simulink library "NNodeTether_cl"  (R2018b)
settings: Solver=VariableStepAuto  StartTime=0.0  StopTime=10.0  RelTol=1e-3
values from neighbouring files (symbols this model uses):
  numNodes = 2    [tether000Test_ts.m]    (also in tether000_init.m = evalin('base',get_param(gcb,'numNodes')))
libraries: nodeDragForce_ul x1, nodeNetBuoyForce_ul x1, nodeSpringDamperForce_ul x1
settings Model: Creator=mcobb  LastModifiedBy=M.Cobb

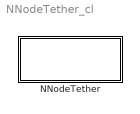
== system NNodeTether_cl ==
  NNodeTether : Subsystem

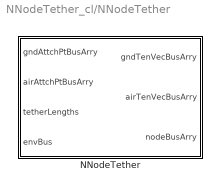
== system NNodeTether_cl/NNodeTether ==
  NNodeTether : Subsystem  mask{thr=0, flowDensity=10, gravity=0}
      mask prompts: thr "Tether Structure"; flowDensity "Fluid Density"; gravity "Gravitational Acceleration"

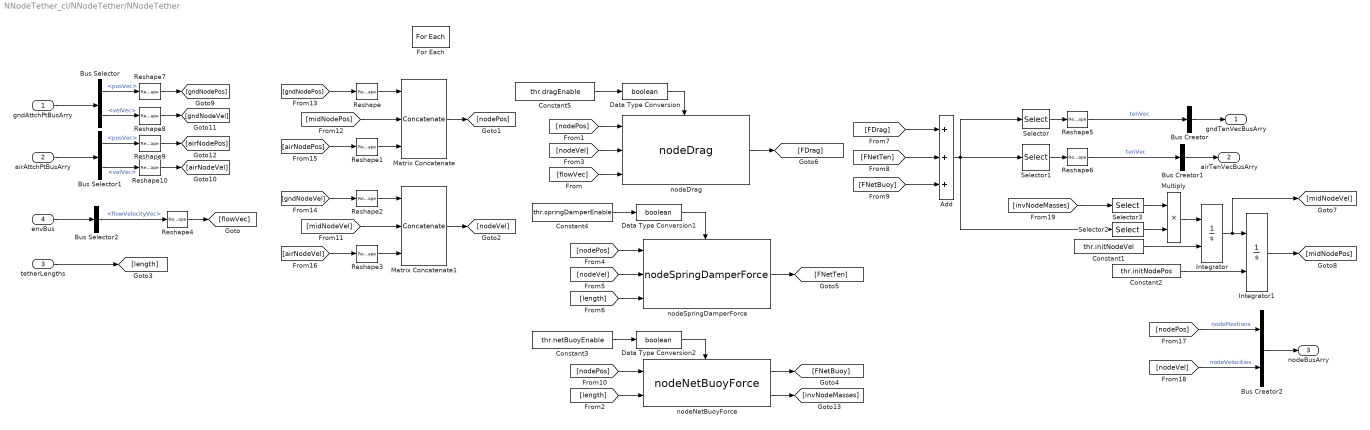
== system NNodeTether_cl/NNodeTether/NNodeTether ==
  gndAttchPtBusArry : Inport  OutDataTypeStr=Bus: thrAttachPtKinematicsBus  Partition=on  PartitionDimension=1  PartitionWidth=1  PartitionOffset=0
  airAttchPtBusArry : Inport  Port=2  OutDataTypeStr=Bus: thrAttachPtKinematicsBus  Partition=on  PartitionDimension=1  PartitionWidth=1  PartitionOffset=0
  tetherLengths : Inport  Port=3  Partition=on  PartitionDimension=1  PartitionWidth=1  PartitionOffset=0
  envBus : Inport  Port=4  OutDataTypeStr=Bus: envBus
  Add : Sum  Inputs=3
  Bus Creator : BusCreator  Inputs=1  OutDataTypeStr=Bus: thrTenVecBus  NonVirtualBus=on
  Bus Creator1 : BusCreator  Inputs=1  OutDataTypeStr=Bus: thrTenVecBus  NonVirtualBus=on
  Bus Creator2 : BusCreator  Inputs=2  OutDataTypeStr=Bus: thrNodeBus  NonVirtualBus=on
  Bus Selector : BusSelector  OutputSignals=posVec,velVec
  Bus Selector1 : BusSelector  OutputSignals=posVec,velVec
  Bus Selector2 : BusSelector  OutputSignals=flowVelocityVec
  Constant1 : Constant  Value=thr.initNodeVel
  Constant2 : Constant  Value=thr.initNodePos
  Constant3 : Constant  Value=thr.netBuoyEnable
  Constant4 : Constant  Value=thr.springDamperEnable
  Constant5 : Constant  Value=thr.dragEnable
  Data Type Conversion : DataTypeConversion  OutDataTypeStr=boolean
  Data Type Conversion1 : DataTypeConversion  OutDataTypeStr=boolean
  Data Type Conversion2 : DataTypeConversion  OutDataTypeStr=boolean
  For Each : ForEach  DisableCoverage=on  IterateSubsysMaskParameter=on,off,off  SubsysMaskParameterIterationDimension=2,1,1  IndexMode=One-based
  Integrator : Integrator  InitialConditionSource=external
  Integrator1 : Integrator  InitialConditionSource=external
  Matrix Concatenate : Concatenate  NumInputs=3  Mode=Multidimensional array  ConcatenateDimension=2
  Matrix Concatenate1 : Concatenate  NumInputs=3  Mode=Multidimensional array  ConcatenateDimension=2
  Multiply : Product
  Reshape{,1..10} (11 alike) : Reshape  OutputDimensionality=Column vector (2-D)
  Selector : Selector  NumberOfDimensions=2  InputPortWidth=3  IndexOptions=Select all,Index vector (dialog)  Indices=[1 3],1  OutputSizes=1,1
  Selector1 : Selector  NumberOfDimensions=2  InputPortWidth=3  IndexOptions=Select all,Starting index (dialog)  Indices=[1 3],numNodes  OutputSizes=1,1
  Selector2 : Selector  NumberOfDimensions=2  InputPortWidth=3  IndexOptions=Select all,Index vector (dialog)  Indices=[1 3],2:numNodes-1  OutputSizes=1,1
  Selector3 : Selector  NumberOfDimensions=2  InputPortWidth=3  IndexOptions=Select all,Index vector (dialog)  Indices=[1 3],2:numNodes-1  OutputSizes=1,1
  nodeDrag : nodeDragForce_ul/nodeDrag  flowDensity=flowDensity  thrDiam=thr.diameter  dragCoeff=thr.dragCoeff
  nodeNetBuoyForce : nodeNetBuoyForce_ul/nodeNetBuoyForce  fluidDensity=flowDensity  tetherDensity=thr.density  diameter=thr.diameter  gravity=gravity
  nodeSpringDamperForce : nodeSpringDamperForce_ul/nodeSpringDamperForce  mass=thr.vehicleMass  zeta=thr.dampingRatio  diameter=thr.diameter  youngsMod=thr.youngsMod
  gndTenVecBusArry : Outport  ConcatenationDimension=1
  airTenVecBusArry : Outport  Port=2  ConcatenationDimension=1
  nodeBusArry : Outport  Port=3  ConcatenationDimension=1
  wires:
  [nodePos] -> nodeNetBuoyForce/1
  Selector1/1 -> Reshape6/1
  Add/1 -> Selector1/1, Selector2/1, Selector/1
  Selector/1 -> Reshape5/1
  [FNetBuoy] -> Add/3
  [FDrag] -> Add/1
  [FNetTen] -> Add/2
  nodeDrag/1 -> [FDrag]
  nodeSpringDamperForce/1 -> [FNetTen]
  nodeNetBuoyForce/1 -> [FNetBuoy]
  nodeNetBuoyForce/2 -> [invNodeMasses]
  [length] -> nodeSpringDamperForce/3
  [nodePos] -> nodeSpringDamperForce/1
  [nodeVel] -> nodeSpringDamperForce/2
  [nodeVel] -> nodeDrag/2
  [length] -> nodeNetBuoyForce/2
  [nodePos] -> nodeDrag/1
  [flowVec] -> nodeDrag/3
  Reshape2/1 -> Matrix Concatenate1/1
  Reshape3/1 -> Matrix Concatenate1/3
  Reshape1/1 -> Matrix Concatenate/3
  Reshape/1 -> Matrix Concatenate/1
  [airNodeVel] -> Reshape3/1
  [airNodePos] -> Reshape1/1
  [gndNodeVel] -> Reshape2/1
  [gndNodePos] -> Reshape/1
  Selector2/1 -> Multiply/2
  Integrator/1 -> [midNodeVel], Integrator1/1
  Integrator1/1 -> [midNodePos]
  [midNodeVel] -> Matrix Concatenate1/2
  [midNodePos] -> Matrix Concatenate/2
  Matrix Concatenate/1 -> [nodePos]
  Reshape10/1 -> [airNodeVel]
  airAttchPtBusArry/1 -> Bus Selector1/1
  Bus Selector/2 -> Reshape8/1  "<velVec>"
  envBus/1 -> Bus Selector2/1
  gndAttchPtBusArry/1 -> Bus Selector/1
  tetherLengths/1 -> [length]
  Bus Selector1/1 -> Reshape9/1  "<posVec>"
  Reshape9/1 -> [airNodePos]
  Bus Selector2/1 -> Reshape4/1  "<flowVelocityVec>"
  Reshape7/1 -> [gndNodePos]
  Bus Selector1/2 -> Reshape10/1  "<velVec>"
  Bus Selector/1 -> Reshape7/1  "<posVec>"
  Reshape8/1 -> [gndNodeVel]
  Reshape4/1 -> [flowVec]
  Bus Creator2/1 -> nodeBusArry/1
  Bus Creator/1 -> gndTenVecBusArry/1
  [nodeVel] -> Bus Creator2/2  "nodeVelocities"
  Bus Creator1/1 -> airTenVecBusArry/1
  Reshape6/1 -> Bus Creator1/1  "tenVec"
  Reshape5/1 -> Bus Creator/1  "tenVec"
  [nodePos] -> Bus Creator2/1  "nodePositions"
  Multiply/1 -> Integrator/1
  Data Type Conversion2/1 -> nodeNetBuoyForce/Enable
  Constant3/1 -> Data Type Conversion2/1
  Constant4/1 -> Data Type Conversion1/1
  Data Type Conversion1/1 -> nodeSpringDamperForce/Enable
  Constant5/1 -> Data Type Conversion/1
  Data Type Conversion/1 -> nodeDrag/Enable
  Constant1/1 -> Integrator/2
  Constant2/1 -> Integrator1/2
  Selector3/1 -> Multiply/1
  [invNodeMasses] -> Selector3/1
  Matrix Concatenate1/1 -> [nodeVel]
